simulink library "Brake_Control_Pressure"  (R2025b)
settings: Solver=VariableStepAuto  StartTime=0.0  StopTime=10.0  RelTol=1e-3
undefined symbols (not defined in the file): Vehicle
Description:
  | Simscape Vehicle Templates Library
  | 
  | Copyright 2018-2025 The MathWorks, Inc.
settings Model: Creator=smiller  LastModifiedBy=smiller
settings OptimizationCC: ReuseModelBlockBuffer=off
settings ModelReferenceCC: EnableRefExpFcnMdlSchedulingChecks=on
settings RTWCC: GPUComputeCapability=3.5

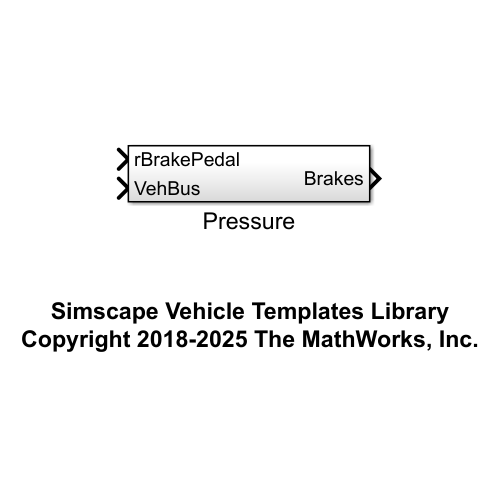
[thumbnail: Simulink's stored preview of the top-level diagram]
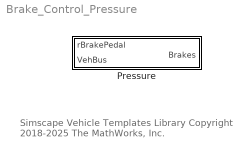
== system Brake_Control_Pressure ==
  note: Simscape Vehicle Templates Library
      | Copyright 2018-2025 The MathWorks, Inc.
  Pressure : Subsystem  VariantControl=Pressure

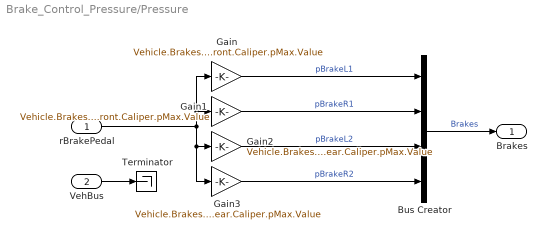
== system Brake_Control_Pressure/Pressure ==
  rBrakePedal : Inport
  VehBus : Inport  Port=2
  Bus Creator : BusCreator  Inputs=4
  Gain : Gain  Gain=Vehicle.Brakes.Front.Caliper.pMax.Value
  Gain1 : Gain  Gain=Vehicle.Brakes.Front.Caliper.pMax.Value
  Gain2 : Gain  Gain=Vehicle.Brakes.Rear.Caliper.pMax.Value
  Gain3 : Gain  Gain=Vehicle.Brakes.Rear.Caliper.pMax.Value
  Terminator : Terminator
  Brakes : Outport  VectorParamsAs1DForOutWhenUnconnected=off
  wires:
  Gain3/1 -> Bus Creator/4  "pBrakeR2"
  Gain2/1 -> Bus Creator/3  "pBrakeL2"
  Gain1/1 -> Bus Creator/2  "pBrakeR1"
  Gain/1 -> Bus Creator/1  "pBrakeL1"
  Bus Creator/1 -> Brakes/1  "Brakes"
  VehBus/1 -> Terminator/1
  rBrakePedal/1 -> Gain2/1, Gain3/1, Gain1/1, Gain/1
